simulink library "BFDAMP_MASTER"  (Simulink 8.5)
settings: Solver=ode45  StartTime=0.0  StopTime=10.0  RelTol=1e-3
libraries: cdsEpicsOut x36, cdsTP x18, cdsFiltCtrl x12, cdsFilt x12, cdsEpicsIn x7, cdsRms x6, cdsMuxMatrix x2, cdsEpicsBinIn x1, cdsFunctionCall x1, SIXOSEM_F_WD_AC_MASTER x1
(part 1 of 3)
settings Model: Creator=controls  LastModifiedBy=controls

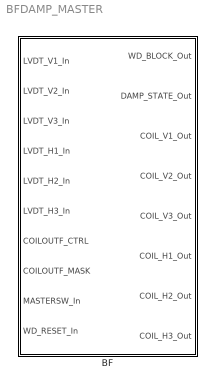
== system BFDAMP_MASTER ==
  BF : Subsystem  Description=SIXOSEMSTAGE_FACE_MASTER

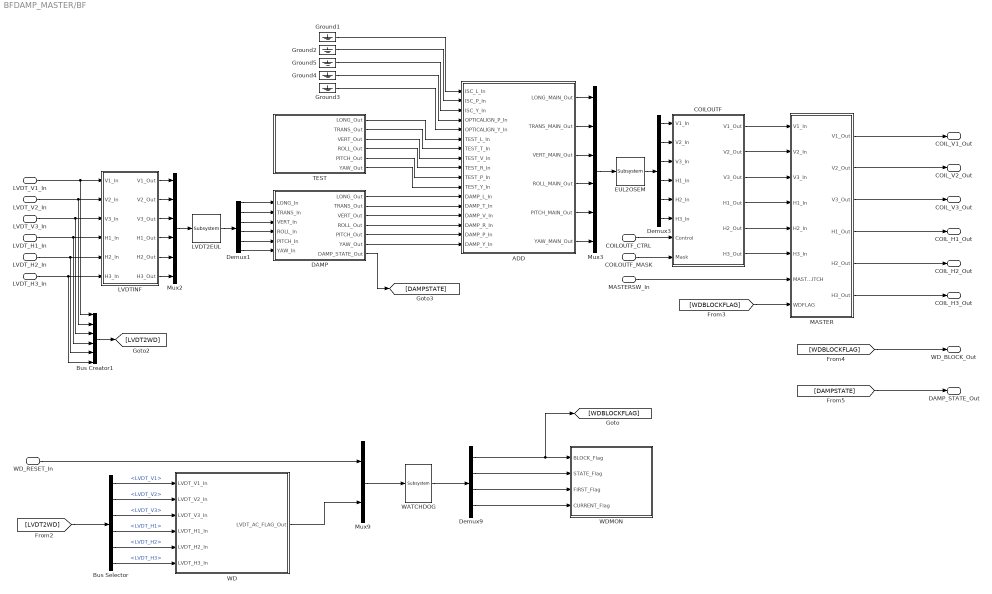
== system BFDAMP_MASTER/BF ==
  LVDT_V1_In : Inport
  LVDT_V2_In : Inport  Port=2
  LVDT_V3_In : Inport  Port=3
  LVDT_H1_In : Inport  Port=4
  LVDT_H2_In : Inport  Port=5
  LVDT_H3_In : Inport  Port=6
  COILOUTF_CTRL : Inport  Port=7
  COILOUTF_MASK : Inport  Port=8
  MASTERSW_In : Inport  Port=9
  WD_RESET_In : Inport  Port=10
  ADD : Subsystem
  Bus Creator1 : BusCreator  Inputs='LVDT_H1','LVDT_H2','LVDT_H3','LVDT_V1','LVDT_V2','LVDT_V3'
  Bus Selector : BusSelector  OutputSignals=LVDT_V1,LVDT_V2,LVDT_V3,LVDT_H1,LVDT_H2,LVDT_H3
  COILOUTF : Subsystem
  DAMP : Subsystem
  Demux1 : Demux  Outputs=6
  Demux3 : Demux  Outputs=6
  Demux9 : Demux
  EUL2OSEM : cdsMuxMatrix/Subsystem  Tag=cdsMuxMatrix  Description=Any size matrix. Inputs and outputs must be connected using Mux and Demux parts.
      settings: AttributesFormatString=%<Tag>
  Ground{1..5} (5 alike) : Ground
  LVDT2EUL : cdsMuxMatrix/Subsystem  Tag=cdsMuxMatrix  Description=Any size matrix. Inputs and outputs must be connected using Mux and Demux parts.
      settings: AttributesFormatString=%<Tag>
  LVDTINF : Subsystem
  MASTER : Subsystem
  Mux2 : Mux  Inputs=6
  Mux3 : Mux  Inputs=6
  Mux9 : Mux  Inputs=2
  TEST : Subsystem
  WATCHDOG : cdsFunctionCall/Subsystem  Tag=cdsFunctionCall  Description=inline OSEMWATCHDOG /opt/rtcds/userapps/release/vis/common/src/WATCHDOG.c
      settings: AttributesFormatString=%<Tag>\n%<Description>
  WD : Subsystem
  WDMON : Subsystem
  WD_BLOCK_Out : Outport
  DAMP_STATE_Out : Outport  Port=2
  COIL_V1_Out : Outport  Port=3
  COIL_V2_Out : Outport  Port=4
  COIL_V3_Out : Outport  Port=5
  COIL_H1_Out : Outport  Port=6
  COIL_H2_Out : Outport  Port=7
  COIL_H3_Out : Outport  Port=8
  wires:
  LVDTINF/1(V1_Out) -> Mux2/1
  WATCHDOG/1 -> Demux9/1
  Mux9/1 -> WATCHDOG/1
  Demux9/4 -> WDMON/4(CURRENT_Flag)
  Demux9/3 -> WDMON/3(FIRST_Flag)
  Demux9/2 -> WDMON/2(STATE_Flag)
  Demux9/1 -> WDMON/1(BLOCK_Flag), [WDBLOCKFLAG]
  [LVDT2WD] -> Bus Selector/1
  Bus Creator1/1 -> [LVDT2WD]
  LVDT_V1_In/1 -> Bus Creator1/1, LVDTINF/1(V1_In)
  [WDBLOCKFLAG] -> MASTER/8(WDFLAG)
  [WDBLOCKFLAG] -> WD_BLOCK_Out/1
  DAMP/7(DAMP_STATE_Out) -> [DAMPSTATE]
  [DAMPSTATE] -> DAMP_STATE_Out/1
  MASTERSW_In/1 -> MASTER/7(MASTERSWITCH)
  COILOUTF_MASK/1 -> COILOUTF/8(Mask)
  COILOUTF_CTRL/1 -> COILOUTF/7(Control)
  WD/1(LVDT_AC_FLAG_Out) -> Mux9/2
  WD_RESET_In/1 -> Mux9/1
  LVDT_V2_In/1 -> Bus Creator1/2, LVDTINF/2(V2_In)
  LVDT_V3_In/1 -> Bus Creator1/3, LVDTINF/3(V3_In)
  LVDTINF/2(V2_Out) -> Mux2/2
  LVDTINF/3(V3_Out) -> Mux2/3
  LVDTINF/5(H2_Out) -> Mux2/5
  LVDTINF/6(H3_Out) -> Mux2/6
  LVDTINF/4(H1_Out) -> Mux2/4
  LVDT_H1_In/1 -> Bus Creator1/4, LVDTINF/4(H1_In)
  LVDT_H2_In/1 -> Bus Creator1/5, LVDTINF/5(H2_In)
  LVDT_H3_In/1 -> Bus Creator1/6, LVDTINF/6(H3_In)
  Mux2/1 -> LVDT2EUL/1
  LVDT2EUL/1 -> Demux1/1
  Demux1/3 -> DAMP/3(VERT_In)
  Demux1/2 -> DAMP/2(TRANS_In)
  Demux1/4 -> DAMP/4(ROLL_In)
  Demux1/1 -> DAMP/1(LONG_In)
  Demux1/5 -> DAMP/5(PITCH_In)
  Demux1/6 -> DAMP/6(YAW_In)
  Mux3/1 -> EUL2OSEM/1
  EUL2OSEM/1 -> Demux3/1
  ADD/1(LONG_MAIN_Out) -> Mux3/1
  ADD/2(TRANS_MAIN_Out) -> Mux3/2
  ADD/3(VERT_MAIN_Out) -> Mux3/3
  ADD/4(ROLL_MAIN_Out) -> Mux3/4
  ADD/5(PITCH_MAIN_Out) -> Mux3/5
  ADD/6(YAW_MAIN_Out) -> Mux3/6
  Demux3/6 -> COILOUTF/6(H3_In)
  Demux3/2 -> COILOUTF/2(V2_In)
  Demux3/3 -> COILOUTF/3(V3_In)
  Demux3/1 -> COILOUTF/1(V1_In)
  Demux3/5 -> COILOUTF/5(H2_In)
  Demux3/4 -> COILOUTF/4(H1_In)
  COILOUTF/4(H1_Out) -> MASTER/4(H1_In)
  COILOUTF/6(H3_Out) -> MASTER/6(H3_In)
  COILOUTF/5(H2_Out) -> MASTER/5(H2_In)
  COILOUTF/3(V3_Out) -> MASTER/3(V3_In)
  COILOUTF/2(V2_Out) -> MASTER/2(V2_In)
  COILOUTF/1(V1_Out) -> MASTER/1(V1_In)
  MASTER/1(V1_Out) -> COIL_V1_Out/1
  MASTER/3(V3_Out) -> COIL_V3_Out/1
  MASTER/2(V2_Out) -> COIL_V2_Out/1
  MASTER/6(H3_Out) -> COIL_H3_Out/1
  MASTER/4(H1_Out) -> COIL_H1_Out/1
  MASTER/5(H2_Out) -> COIL_H2_Out/1
  Ground3/1 -> ADD/5(OPTICALIGN_Y_In)
  Ground4/1 -> ADD/4(OPTICALIGN_P_In)
  Ground5/1 -> ADD/3(ISC_Y_In)
  Ground2/1 -> ADD/2(ISC_P_In)
  Ground1/1 -> ADD/1(ISC_L_In)
  TEST/6(YAW_Out) -> ADD/11(TEST_Y_In)
  TEST/5(PITCH_Out) -> ADD/10(TEST_P_In)
  TEST/4(ROLL_Out) -> ADD/9(TEST_R_In)
  TEST/3(VERT_Out) -> ADD/8(TEST_V_In)
  TEST/2(TRANS_Out) -> ADD/7(TEST_T_In)
  TEST/1(LONG_Out) -> ADD/6(TEST_L_In)
  DAMP/4(ROLL_Out) -> ADD/15(DAMP_R_In)
  DAMP/3(VERT_Out) -> ADD/14(DAMP_V_In)
  DAMP/5(PITCH_Out) -> ADD/16(DAMP_P_In)
  DAMP/6(YAW_Out) -> ADD/17(DAMP_Y_In)
  DAMP/2(TRANS_Out) -> ADD/13(DAMP_T_In)
  DAMP/1(LONG_Out) -> ADD/12(DAMP_L_In)
  Bus Selector/4 -> WD/4(LVDT_H1_In)  "<LVDT_H1>"
  Bus Selector/5 -> WD/5(LVDT_H2_In)  "<LVDT_H2>"
  Bus Selector/6 -> WD/6(LVDT_H3_In)  "<LVDT_H3>"
  Bus Selector/1 -> WD/1(LVDT_V1_In)  "<LVDT_V1>"
  Bus Selector/2 -> WD/2(LVDT_V2_In)  "<LVDT_V2>"
  Bus Selector/3 -> WD/3(LVDT_V3_In)  "<LVDT_V3>"

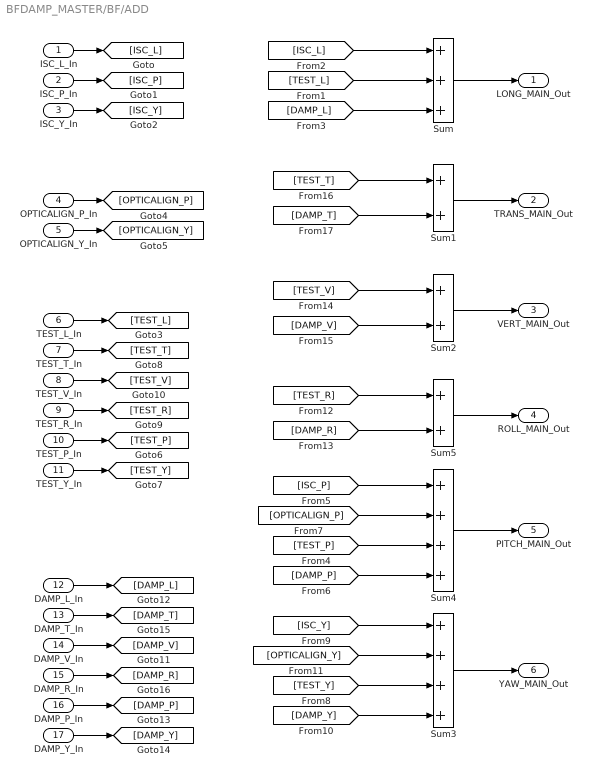
== system BFDAMP_MASTER/BF/ADD ==
  ISC_L_In : Inport
  ISC_P_In : Inport  Port=2
  ISC_Y_In : Inport  Port=3
  OPTICALIGN_P_In : Inport  Port=4
  OPTICALIGN_Y_In : Inport  Port=5
  TEST_L_In : Inport  Port=6
  TEST_T_In : Inport  Port=7
  TEST_V_In : Inport  Port=8
  TEST_R_In : Inport  Port=9
  TEST_P_In : Inport  Port=10
  TEST_Y_In : Inport  Port=11
  DAMP_L_In : Inport  Port=12
  DAMP_T_In : Inport  Port=13
  DAMP_V_In : Inport  Port=14
  DAMP_R_In : Inport  Port=15
  DAMP_P_In : Inport  Port=16
  DAMP_Y_In : Inport  Port=17
  Sum : Sum  Inputs=+++
  Sum1 : Sum
  Sum2 : Sum
  Sum3 : Sum  Inputs=++++
  Sum4 : Sum  Inputs=++++
  Sum5 : Sum
  LONG_MAIN_Out : Outport
  TRANS_MAIN_Out : Outport  Port=2
  VERT_MAIN_Out : Outport  Port=3
  ROLL_MAIN_Out : Outport  Port=4
  PITCH_MAIN_Out : Outport  Port=5
  YAW_MAIN_Out : Outport  Port=6
  wires:
  [DAMP_V] -> Sum2/2
  [TEST_V] -> Sum2/1
  [DAMP_T] -> Sum1/2
  [TEST_T] -> Sum1/1
  [DAMP_R] -> Sum5/2
  [TEST_R] -> Sum5/1
  [DAMP_Y] -> Sum3/4
  [TEST_Y] -> Sum3/3
  [OPTICALIGN_Y] -> Sum3/2
  [ISC_Y] -> Sum3/1
  [DAMP_P] -> Sum4/4
  [TEST_P] -> Sum4/3
  [OPTICALIGN_P] -> Sum4/2
  [ISC_P] -> Sum4/1
  DAMP_Y_In/1 -> [DAMP_Y]
  DAMP_P_In/1 -> [DAMP_P]
  DAMP_R_In/1 -> [DAMP_R]
  DAMP_V_In/1 -> [DAMP_V]
  DAMP_T_In/1 -> [DAMP_T]
  DAMP_L_In/1 -> [DAMP_L]
  TEST_Y_In/1 -> [TEST_Y]
  TEST_P_In/1 -> [TEST_P]
  TEST_R_In/1 -> [TEST_R]
  TEST_V_In/1 -> [TEST_V]
  TEST_T_In/1 -> [TEST_T]
  TEST_L_In/1 -> [TEST_L]
  ISC_Y_In/1 -> [ISC_Y]
  ISC_P_In/1 -> [ISC_P]
  ISC_L_In/1 -> [ISC_L]
  OPTICALIGN_Y_In/1 -> [OPTICALIGN_Y]
  OPTICALIGN_P_In/1 -> [OPTICALIGN_P]
  Sum1/1 -> TRANS_MAIN_Out/1
  Sum2/1 -> VERT_MAIN_Out/1
  Sum5/1 -> ROLL_MAIN_Out/1
  [DAMP_L] -> Sum/3
  [TEST_L] -> Sum/2
  [ISC_L] -> Sum/1
  Sum/1 -> LONG_MAIN_Out/1
  Sum3/1 -> YAW_MAIN_Out/1
  Sum4/1 -> PITCH_MAIN_Out/1

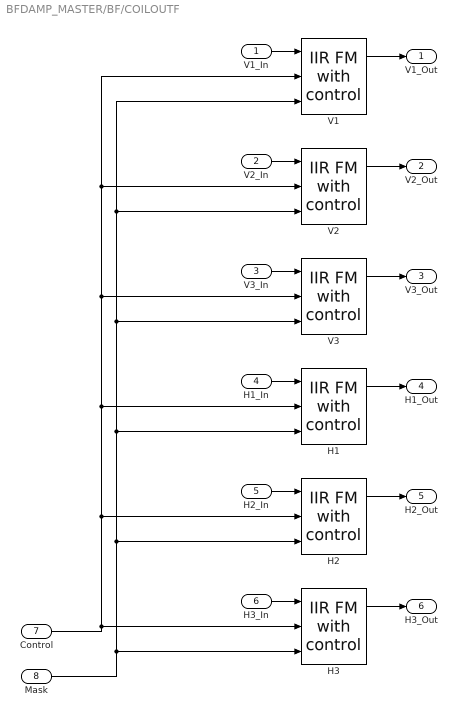
== system BFDAMP_MASTER/BF/COILOUTF ==
  V1_In : Inport
  V2_In : Inport  Port=2
  V3_In : Inport  Port=3
  H1_In : Inport  Port=4
  H2_In : Inport  Port=5
  H3_In : Inport  Port=6
  Control : Inport  Port=7
  Mask : Inport  Port=8
  H1 : cdsFiltCtrl/IIR FM with control  Tag=cdsFiltCtrl  Description=|
      | cdsFiltCntrl is the standard IIR filter module (exactly the same as cdsFilt) but with added control data output 'Ctrl'. Filter module digital signal output appears on the first output, which is called 'Val'. 'Ctrl' output has a bit pattern encoding the state of filter's on/off switches (FM1 through FM10). The bit values are:
      |                                                                                                                                                                                                                                                                                                                                       
      | module 	hex	dec                                                                                                                                                                                                                                                                                                                       
      | -----------------------                                                                                                                                                                                                                                                                                                               
      | FM1	0x20                    32                                                                                                                                                                                                                                                                                                        
      | FM2	0x80                     128                                                                                                                                                                                                                                                                                                      
      | FM3	0x200                   512                                                                                                                                                                                                                                                                                                       
      | FM4	0x800                   2048                                                                                                                                                                                                                                                                                                      
      | FM5	0x2000                 8192                                                                                                                                                                                                                                                                                                       
      | FM6	0x8000                 32768                                                                                                                                                                                                                                                                                                      
      | FM7	0x20000                131072                                                                                                                                                                                                                                                                                                     
      | FM8	0x80000                 524288                                                                                                                                                                                                                                                                                                    
      | FM9	0x200000               2097152                                                                                                                                                                                                                                                                                                    
      | FM10	0x800000               8388608                                                                                                                                                                                                                                                                                                   
      |                                                                                                                                                                                                                                                                                                                                       
      | This bit data can be used to drive some other switches or it can be output using a binary I/O module.
      settings: AttributesFormatString=%<Tag>
  H2 : cdsFiltCtrl/IIR FM with control  Tag=cdsFiltCtrl  Description=|
      | cdsFiltCntrl is the standard IIR filter module (exactly the same as cdsFilt) but with added control data output 'Ctrl'. Filter module digital signal output appears on the first output, which is called 'Val'. 'Ctrl' output has a bit pattern encoding the state of filter's on/off switches (FM1 through FM10). The bit values are:
      |                                                                                                                                                                                                                                                                                                                                       
      | module 	hex	dec                                                                                                                                                                                                                                                                                                                       
      | -----------------------                                                                                                                                                                                                                                                                                                               
      | FM1	0x20                    32                                                                                                                                                                                                                                                                                                        
      | FM2	0x80                     128                                                                                                                                                                                                                                                                                                      
      | FM3	0x200                   512                                                                                                                                                                                                                                                                                                       
      | FM4	0x800                   2048                                                                                                                                                                                                                                                                                                      
      | FM5	0x2000                 8192                                                                                                                                                                                                                                                                                                       
      | FM6	0x8000                 32768                                                                                                                                                                                                                                                                                                      
      | FM7	0x20000                131072                                                                                                                                                                                                                                                                                                     
      | FM8	0x80000                 524288                                                                                                                                                                                                                                                                                                    
      | FM9	0x200000               2097152                                                                                                                                                                                                                                                                                                    
      | FM10	0x800000               8388608                                                                                                                                                                                                                                                                                                   
      |                                                                                                                                                                                                                                                                                                                                       
      | This bit data can be used to drive some other switches or it can be output using a binary I/O module.
      settings: AttributesFormatString=%<Tag>
  H3 : cdsFiltCtrl/IIR FM with control  Tag=cdsFiltCtrl  Description=|
      | cdsFiltCntrl is the standard IIR filter module (exactly the same as cdsFilt) but with added control data output 'Ctrl'. Filter module digital signal output appears on the first output, which is called 'Val'. 'Ctrl' output has a bit pattern encoding the state of filter's on/off switches (FM1 through FM10). The bit values are:
      |                                                                                                                                                                                                                                                                                                                                       
      | module 	hex	dec                                                                                                                                                                                                                                                                                                                       
      | -----------------------                                                                                                                                                                                                                                                                                                               
      | FM1	0x20                    32                                                                                                                                                                                                                                                                                                        
      | FM2	0x80                     128                                                                                                                                                                                                                                                                                                      
      | FM3	0x200                   512                                                                                                                                                                                                                                                                                                       
      | FM4	0x800                   2048                                                                                                                                                                                                                                                                                                      
      | FM5	0x2000                 8192                                                                                                                                                                                                                                                                                                       
      | FM6	0x8000                 32768                                                                                                                                                                                                                                                                                                      
      | FM7	0x20000                131072                                                                                                                                                                                                                                                                                                     
      | FM8	0x80000                 524288                                                                                                                                                                                                                                                                                                    
      | FM9	0x200000               2097152                                                                                                                                                                                                                                                                                                    
      | FM10	0x800000               8388608                                                                                                                                                                                                                                                                                                   
      |                                                                                                                                                                                                                                                                                                                                       
      | This bit data can be used to drive some other switches or it can be output using a binary I/O module.
      settings: AttributesFormatString=%<Tag>
  V1 : cdsFiltCtrl/IIR FM with control  Tag=cdsFiltCtrl  Description=|
      | cdsFiltCntrl is the standard IIR filter module (exactly the same as cdsFilt) but with added control data output 'Ctrl'. Filter module digital signal output appears on the first output, which is called 'Val'. 'Ctrl' output has a bit pattern encoding the state of filter's on/off switches (FM1 through FM10). The bit values are:
      |                                                                                                                                                                                                                                                                                                                                       
      | module 	hex	dec                                                                                                                                                                                                                                                                                                                       
      | -----------------------                                                                                                                                                                                                                                                                                                               
      | FM1	0x20                    32                                                                                                                                                                                                                                                                                                        
      | FM2	0x80                     128                                                                                                                                                                                                                                                                                                      
      | FM3	0x200                   512                                                                                                                                                                                                                                                                                                       
      | FM4	0x800                   2048                                                                                                                                                                                                                                                                                                      
      | FM5	0x2000                 8192                                                                                                                                                                                                                                                                                                       
      | FM6	0x8000                 32768                                                                                                                                                                                                                                                                                                      
      | FM7	0x20000                131072                                                                                                                                                                                                                                                                                                     
      | FM8	0x80000                 524288                                                                                                                                                                                                                                                                                                    
      | FM9	0x200000               2097152                                                                                                                                                                                                                                                                                                    
      | FM10	0x800000               8388608                                                                                                                                                                                                                                                                                                   
      |                                                                                                                                                                                                                                                                                                                                       
      | This bit data can be used to drive some other switches or it can be output using a binary I/O module.
      settings: AttributesFormatString=%<Tag>
  V2 : cdsFiltCtrl/IIR FM with control  Tag=cdsFiltCtrl  Description=|
      | cdsFiltCntrl is the standard IIR filter module (exactly the same as cdsFilt) but with added control data output 'Ctrl'. Filter module digital signal output appears on the first output, which is called 'Val'. 'Ctrl' output has a bit pattern encoding the state of filter's on/off switches (FM1 through FM10). The bit values are:
      |                                                                                                                                                                                                                                                                                                                                       
      | module 	hex	dec                                                                                                                                                                                                                                                                                                                       
      | -----------------------                                                                                                                                                                                                                                                                                                               
      | FM1	0x20                    32                                                                                                                                                                                                                                                                                                        
      | FM2	0x80                     128                                                                                                                                                                                                                                                                                                      
      | FM3	0x200                   512                                                                                                                                                                                                                                                                                                       
      | FM4	0x800                   2048                                                                                                                                                                                                                                                                                                      
      | FM5	0x2000                 8192                                                                                                                                                                                                                                                                                                       
      | FM6	0x8000                 32768                                                                                                                                                                                                                                                                                                      
      | FM7	0x20000                131072                                                                                                                                                                                                                                                                                                     
      | FM8	0x80000                 524288                                                                                                                                                                                                                                                                                                    
      | FM9	0x200000               2097152                                                                                                                                                                                                                                                                                                    
      | FM10	0x800000               8388608                                                                                                                                                                                                                                                                                                   
      |                                                                                                                                                                                                                                                                                                                                       
      | This bit data can be used to drive some other switches or it can be output using a binary I/O module.
      settings: AttributesFormatString=%<Tag>
  V3 : cdsFiltCtrl/IIR FM with control  Tag=cdsFiltCtrl  Description=|
      | cdsFiltCntrl is the standard IIR filter module (exactly the same as cdsFilt) but with added control data output 'Ctrl'. Filter module digital signal output appears on the first output, which is called 'Val'. 'Ctrl' output has a bit pattern encoding the state of filter's on/off switches (FM1 through FM10). The bit values are:
      |                                                                                                                                                                                                                                                                                                                                       
      | module 	hex	dec                                                                                                                                                                                                                                                                                                                       
      | -----------------------                                                                                                                                                                                                                                                                                                               
      | FM1	0x20                    32                                                                                                                                                                                                                                                                                                        
      | FM2	0x80                     128                                                                                                                                                                                                                                                                                                      
      | FM3	0x200                   512                                                                                                                                                                                                                                                                                                       
      | FM4	0x800                   2048                                                                                                                                                                                                                                                                                                      
      | FM5	0x2000                 8192                                                                                                                                                                                                                                                                                                       
      | FM6	0x8000                 32768                                                                                                                                                                                                                                                                                                      
      | FM7	0x20000                131072                                                                                                                                                                                                                                                                                                     
      | FM8	0x80000                 524288                                                                                                                                                                                                                                                                                                    
      | FM9	0x200000               2097152                                                                                                                                                                                                                                                                                                    
      | FM10	0x800000               8388608                                                                                                                                                                                                                                                                                                   
      |                                                                                                                                                                                                                                                                                                                                       
      | This bit data can be used to drive some other switches or it can be output using a binary I/O module.
      settings: AttributesFormatString=%<Tag>
  V1_Out : Outport
  V2_Out : Outport  Port=2
  V3_Out : Outport  Port=3
  H1_Out : Outport  Port=4
  H2_Out : Outport  Port=5
  H3_Out : Outport  Port=6
  wires:
  Mask/1 -> H3/3, H2/3, H1/3, V3/3, V2/3, V1/3
  Control/1 -> H3/2, H2/2, H1/2, V3/2, V2/2, V1/2
  V1/1 -> V1_Out/1
  V1_In/1 -> V1/1
  V2_In/1 -> V2/1
  V2/1 -> V2_Out/1
  V3_In/1 -> V3/1
  V3/1 -> V3_Out/1
  H1_In/1 -> H1/1
  H1/1 -> H1_Out/1
  H2_In/1 -> H2/1
  H2/1 -> H2_Out/1
  H3_In/1 -> H3/1
  H3/1 -> H3_Out/1
